simulink model "fig2_45_simulink"  (R2021b)
settings: Solver=ode45  StartTime=0.0  StopTime=400  RelTol=1e-3  EnableMultiTasking=on
settings Model: Creator=One Informatic  LastModifiedBy=One Informatic
settings DataIOCC: LimitDataPoints=on  SaveFormat=Array  SignalLoggingSaveFormat=ModelDataLogs  ReturnWorkspaceOutputs=off  SignalLoggingName=sigsOut
settings DebuggingCC: SaveWithParameterizedLinksMsg=none  UnderspecifiedInitializationDetection=Classic  MergeDetectMultiDrivingBlocksExec=none  SignalResolutionControl=TryResolveAllWithWarning  MultiTaskDSMMsg=warning  MultiTaskCondExecSysMsg=none
settings HardwareCC: ProdBitPerPointer=32  ProdBitPerSizeT=32  ProdBitPerPtrDiffT=32  ProdLargestAtomicFloat=None  ProdIntDivRoundTo=Undefined  ProdEndianess=Unspecified  ProdWordSize=32  ProdHWDeviceType=32-bit Generic  TargetUnknown=on
settings ModelReferenceCC: PropagateSignalLabelsOutOfModel=off
settings GRTTargetCC: CombineOutputUpdateFcns=off  GRTInterface=on
settings ConfigComp: CovMetricSettings=dw  CovSaveCumulativeToWorkspaceVar=on  CovSaveSingleToWorkspaceVar=on

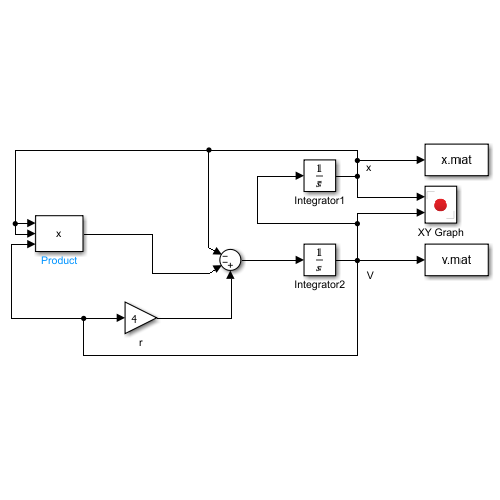
[thumbnail: Simulink's stored preview of the top-level diagram]
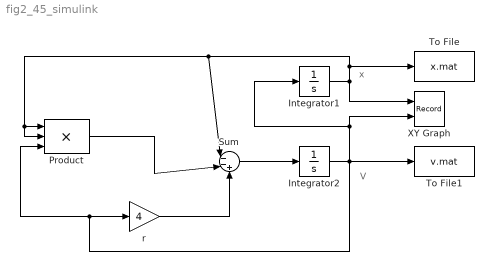
== system fig2_45_simulink ==
  note: x
  note: V
  Integrator1 : Integrator  InitialCondition=0.2
  Integrator2 : Integrator  InitialCondition=0.1
  Product : Product  Inputs=3  SaturateOnIntegerOverflow=on  OutDataTypeStr=Inherit: Same as first input
  Sum : Sum  Inputs=|--+  SaturateOnIntegerOverflow=on
  To File : ToFile  Filename=x.mat  MatrixName=x  SampleTime=0.001
  To File1 : ToFile  Filename=v.mat  MatrixName=v  SampleTime=0.001
  XY Graph : Record  FileSettingsInternal="{\"entries\":[{\"content\":{\"excelSettings\":{\"content\":{},\"type\":\"Streamout.ExcelSettings\"}},\"type\":\"Streamout.FileSettingStorage\",\"uuid\":\"a55beb16-261f-430d-98d1-ffd28f0215ee\"}],\"packageUris\":[\"http://schema.mathworks.com/mf0/streamout_blocks/R2020a\"],\"version\":\"1.0\"}"  Layout=[1 1]  SignalsInternal="{\"entries\":[{\"content\":{\"signals\":[{\"content\":{\"blockPath\":[\"h14/XY Graph\"],\"channel\":[],\"dimensions\":[1],\"domain\":\"h14/XY Graph\",\"lineColor\":\"#a2142f\",\"plots\":[1],\"port\":1,\"sid\":[],\"signalID\":116995,\"signalName\":\"XY Graph:1\"},\"type\":\"RecordBlkView.Signal\",\"uuid\":\"b1a125aa-9a51-4877-94ac-8bcd8d53c9ea\"},{\"content\":{\"blockPath\":[\"h14/XY Graph\"],\"channel\":[],\"dimensions\":[1],\"domain\":\"h14/XY Graph\",\"lineColor\":\"#139fff\",\"plots\":[1],\"port\":2,\"sid\":[],\"signalID\":116998,\"signalName\":\"XY Graph:2\"},\"type\":\"RecordBlkView.Signal\",\"uuid\":\"c6ca85c6-868e-4348-9955-bb0779d73344\"}]},\"type\":\"RecordBlkView.InputSignals\",\"uuid\":\"6583f906-9730-46b3-9f15-01dd1196fa31\"}],\"packageUris\":[\"http://schema.mathworks.com/mf0/streamout_blocks/R2020a\"],\"version\":\"1.0\"}"  VisualizationBindings="{\"xyplotplugin\":{\"info\":[{\"series\":[{\"bindingParametersList\":[{\"parameter\":\"X-Axis\",\"signalID\":116995,\"signalName\":\"XY Graph:1\"},{\"parameter\":\"Y-Axis\",\"signalID\":116998,\"signalName\":\"XY Graph:2\"}],\"seriesID\":37356}],\"subplotID\":1}]}}"  CompatibilityTag=XY  st=0.05
  r : Gain  Gain=4  SaturateOnIntegerOverflow=on  OutDataTypeStr=Inherit: Same as input  ParamDataTypeStr=Inherit: Same as input
  wires:
  Sum/1 -> Integrator2/1
  Integrator2/1 -> r/1, Product/3, To File1/1, Integrator1/1, XY Graph/2
  Integrator1/1 -> Sum/1, Product/1, Product/2, To File/1, XY Graph/1
  Product/1 -> Sum/2
  r/1 -> Sum/3
